simulink model "special_points"  (R2022b)
settings: Solver=VariableStepAuto  StartTime=0.0  StopTime=10  RelTol=1e-3
settings Model: Creator=Ivan  LastModifiedBy=anver
settings OptimizationCC: ReuseModelBlockBuffer=on

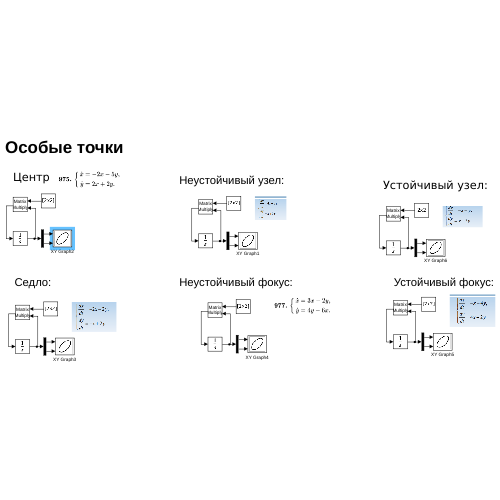
[thumbnail: Simulink's stored preview of the top-level diagram]
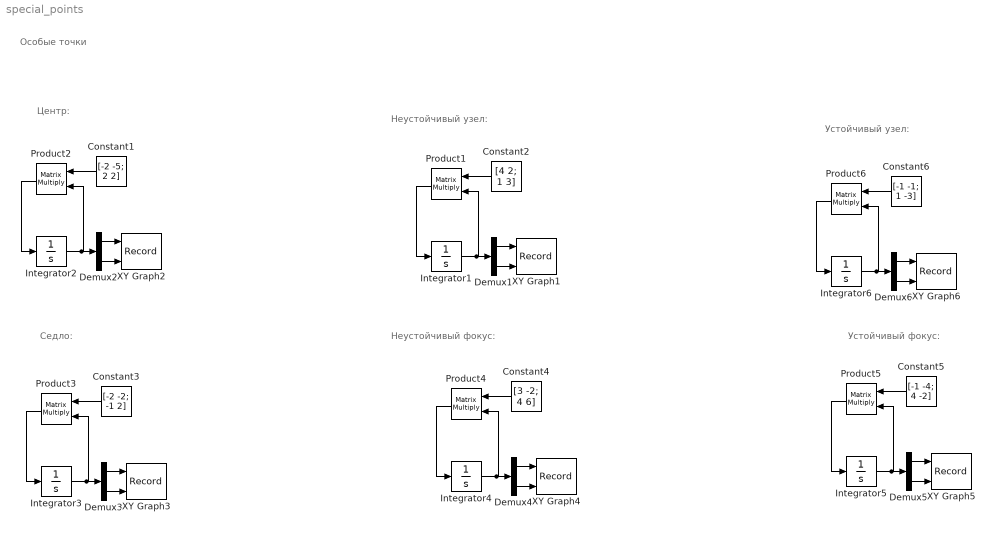
== system special_points ==
  note: Устойчивый узел:
  note: Седло:
  note: Центр:
  note: Особые точки
  note: Неустойчивый фокус:
  note: Неустойчивый узел:
  note: Устойчивый фокус:
  Constant1 : Constant  Value=[-2 -5; 2 2]
  Constant2 : Constant  Value=[4 2; 1 3]
  Constant3 : Constant  Value=[-2 -2; -1 2]
  Constant4 : Constant  Value=[3 -2; 4 6]
  Constant5 : Constant  Value=[-1 -4; 4 -2]
  Constant6 : Constant  Value=[-1 -1; 1 -3]
  Demux{1..6} (6 alike) : Demux  Outputs=2
  Integrator{1..6} (6 alike) : Integrator  InitialCondition=[1; 1]
  Product{1..6} (6 alike) : Product  Multiplication=Matrix(*)
  XY Graph1 : Record  FileSettingsInternal="{\"entries\":[{\"content\":{\"excelSettings\":{\"content\":{},\"type\":\"Streamout.ExcelSettings\"}},\"type\":\"Streamout.FileSettingStorage\",\"uuid\":\"b29d8a9c-392a-4fb2-98d1-ab0fd2f5d560\"}],\"packageUris\":[\"http://schema.mathworks.com/mf0/streamout_blocks/R2020a\"],\"version\":\"1.0\"}"  Layout=[1 1]  SignalsInternal="{\"entries\":[{\"content\":{\"signals\":[{\"content\":{\"blockPath\":[\"specialpoints/XY Graph1\"],\"channel\":[],\"dimensions\":[1],\"domain\":\"specialpoints/XY Graph1\",\"lineColor\":\"#a2142f\",\"plots\":[1],\"port\":1,\"sid\":[\"\"],\"signalID\":67,\"signalName\":\"Demux1:1\"},\"type\":\"RecordBlkView.Signal\",\"uuid\":\"e284521d-6ec3-49b5-a947-304f1478cd59\"},{\"content\":{\"blockPath\":[\"specialpoints/XY Graph1\"],\"channel\":[],\"dimensions\":[1],\"domain\":\"specialpoints/XY Graph1\",\"lineColor\":\"#139fff\",\"plots\":[1],\"port\":2,\"sid\":[\"\"],\"signalID\":71,\"signalName\":\"Demux1:2\"},\"type\":\"RecordBlkView.Signal\",\"uuid\":\"8df6b733-6354-4f83-b4f7-c70068da76a6\"}]},\"type\":\"RecordBlkView.InputSignals\",\"uuid\":\"bb9e6b20-75a7-4c07-86ad-f0d557820732\"}],\"packageUris\":[\"http://schema.mathworks.com/mf0/streamout_blocks/R2020a\"],\"version\":\"1.0\"}"  VisualizationBindings="{\"xyplotplugin\":{\"info\":[{\"series\":[{\"bindingParametersList\":[{\"parameter\":\"X-Axis\",\"signalID\":67,\"signalName\":\"Demux1:1\"},{\"parameter\":\"Y-Axis\",\"signalID\":71,\"signalName\":\"Demux1:2\"}],\"seriesID\":26685}],\"subplotID\":1}]}}"  CompatibilityTag=XY
  XY Graph2 : Record  FileSettingsInternal="{\"entries\":[{\"content\":{\"excelSettings\":{\"content\":{},\"type\":\"Streamout.ExcelSettings\"}},\"type\":\"Streamout.FileSettingStorage\",\"uuid\":\"a0532e12-d950-4453-bbc3-ca59d96ccae8\"}],\"packageUris\":[\"http://schema.mathworks.com/mf0/streamout_blocks/R2020a\"],\"version\":\"1.0\"}"  Layout=[1 1]  SignalsInternal="{\"entries\":[{\"content\":{\"signals\":[{\"content\":{\"blockPath\":[\"specialpoints/XY Graph2\"],\"channel\":[],\"dimensions\":[1],\"domain\":\"specialpoints/XY Graph2\",\"lineColor\":\"#a2142f\",\"plots\":[1],\"port\":1,\"sid\":[\"\"],\"signalID\":59,\"signalName\":\"Demux2:1\"},\"type\":\"RecordBlkView.Signal\",\"uuid\":\"02553b2b-631b-43a1-b492-2037fb39ac76\"},{\"content\":{\"blockPath\":[\"specialpoints/XY Graph2\"],\"channel\":[],\"dimensions\":[1],\"domain\":\"specialpoints/XY Graph2\",\"lineColor\":\"#139fff\",\"plots\":[1],\"port\":2,\"sid\":[\"\"],\"signalID\":63,\"signalName\":\"Demux2:2\"},\"type\":\"RecordBlkView.Signal\",\"uuid\":\"8bd99721-c510-42f4-8a47-9157c50785ae\"}]},\"type\":\"RecordBlkView.InputSignals\",\"uuid\":\"8468d6b2-b3e3-4423-a976-07fda8fce5e6\"}],\"packageUris\":[\"http://schema.mathworks.com/mf0/streamout_blocks/R2020a\"],\"version\":\"1.0\"}"  VisualizationBindings="{\"xyplotplugin\":{\"info\":[{\"series\":[{\"bindingParametersList\":[{\"parameter\":\"X-Axis\",\"signalID\":59,\"signalName\":\"Demux2:1\"},{\"parameter\":\"Y-Axis\",\"signalID\":63,\"signalName\":\"Demux2:2\"}],\"seriesID\":13331}],\"subplotID\":1}]}}"  CompatibilityTag=XY
  XY Graph3 : Record  FileSettingsInternal="{\"entries\":[{\"content\":{\"excelSettings\":{\"content\":{},\"type\":\"Streamout.ExcelSettings\"}},\"type\":\"Streamout.FileSettingStorage\",\"uuid\":\"69cbb6f6-f3a5-44cd-92ef-4036cbebcdd5\"}],\"packageUris\":[\"http://schema.mathworks.com/mf0/streamout_blocks/R2020a\"],\"version\":\"1.0\"}"  Layout=[1 1]  SignalsInternal="{\"entries\":[{\"content\":{\"signals\":[{\"content\":{\"blockPath\":[\"specialpoints/XY Graph3\"],\"channel\":[],\"dimensions\":[1],\"domain\":\"specialpoints/XY Graph3\",\"lineColor\":\"#a2142f\",\"plots\":[1],\"port\":1,\"sid\":[\"\"],\"signalID\":75,\"signalName\":\"Demux3:1\"},\"type\":\"RecordBlkView.Signal\",\"uuid\":\"47cecb95-6076-4ee7-86e1-f1b5dc16acf8\"},{\"content\":{\"blockPath\":[\"specialpoints/XY Graph3\"],\"channel\":[],\"dimensions\":[1],\"domain\":\"specialpoints/XY Graph3\",\"lineColor\":\"#139fff\",\"plots\":[1],\"port\":2,\"sid\":[\"\"],\"signalID\":79,\"signalName\":\"Demux3:2\"},\"type\":\"RecordBlkView.Signal\",\"uuid\":\"91964f3b-7724-463e-8b5d-57be4e640c57\"}]},\"type\":\"RecordBlkView.InputSignals\",\"uuid\":\"1ea9a202-36d1-423e-b5ef-d386424ed832\"}],\"packageUris\":[\"http://schema.mathworks.com/mf0/streamout_blocks/R2020a\"],\"version\":\"1.0\"}"  VisualizationBindings="{\"xyplotplugin\":{\"info\":[{\"series\":[{\"bindingParametersList\":[{\"parameter\":\"X-Axis\",\"signalID\":75,\"signalName\":\"Demux3:1\"},{\"parameter\":\"Y-Axis\",\"signalID\":79,\"signalName\":\"Demux3:2\"}],\"seriesID\":54321}],\"subplotID\":1}]}}"  CompatibilityTag=XY
  XY Graph4 : Record  FileSettingsInternal="{\"entries\":[{\"content\":{\"excelSettings\":{\"content\":{},\"type\":\"Streamout.ExcelSettings\"}},\"type\":\"Streamout.FileSettingStorage\",\"uuid\":\"88a36fd6-7621-4d16-9cb3-468432706825\"}],\"packageUris\":[\"http://schema.mathworks.com/mf0/streamout_blocks/R2020a\"],\"version\":\"1.0\"}"  Layout=[1 1]  SignalsInternal="{\"entries\":[{\"content\":{\"signals\":[{\"content\":{\"blockPath\":[\"specialpoints/XY Graph4\"],\"channel\":[],\"dimensions\":[1],\"domain\":\"specialpoints/XY Graph4\",\"lineColor\":\"#a2142f\",\"plots\":[1],\"port\":1,\"sid\":[\"\"],\"signalID\":83,\"signalName\":\"Demux4:1\"},\"type\":\"RecordBlkView.Signal\",\"uuid\":\"77b31cb0-8e9b-42f2-81eb-f84cb2f67803\"},{\"content\":{\"blockPath\":[\"specialpoints/XY Graph4\"],\"channel\":[],\"dimensions\":[1],\"domain\":\"specialpoints/XY Graph4\",\"lineColor\":\"#139fff\",\"plots\":[1],\"port\":2,\"sid\":[\"\"],\"signalID\":87,\"signalName\":\"Demux4:2\"},\"type\":\"RecordBlkView.Signal\",\"uuid\":\"21fa5dc8-c382-464e-aa4c-53efbbb9609e\"}]},\"type\":\"RecordBlkView.InputSignals\",\"uuid\":\"7114cbdf-c82f-41cb-8a52-ea1fd9a40c1c\"}],\"packageUris\":[\"http://schema.mathworks.com/mf0/streamout_blocks/R2020a\"],\"version\":\"1.0\"}"  VisualizationBindings="{\"xyplotplugin\":{\"info\":[{\"series\":[{\"bindingParametersList\":[{\"parameter\":\"X-Axis\",\"signalID\":83,\"signalName\":\"Demux4:1\"},{\"parameter\":\"Y-Axis\",\"signalID\":87,\"signalName\":\"Demux4:2\"}],\"seriesID\":54038}],\"subplotID\":1}]}}"  CompatibilityTag=XY
  XY Graph5 : Record  FileSettingsInternal="{\"entries\":[{\"content\":{\"excelSettings\":{\"content\":{},\"type\":\"Streamout.ExcelSettings\"}},\"type\":\"Streamout.FileSettingStorage\",\"uuid\":\"fc638fc8-ea17-4822-ae91-b9c87cfefd68\"}],\"packageUris\":[\"http://schema.mathworks.com/mf0/streamout_blocks/R2020a\"],\"version\":\"1.0\"}"  Layout=[1 1]  SignalsInternal="{\"entries\":[{\"content\":{\"signals\":[{\"content\":{\"blockPath\":[\"specialpoints/XY Graph5\"],\"channel\":[],\"dimensions\":[1],\"domain\":\"specialpoints/XY Graph5\",\"lineColor\":\"#a2142f\",\"plots\":[1],\"port\":1,\"sid\":[\"\"],\"signalID\":91,\"signalName\":\"Demux5:1\"},\"type\":\"RecordBlkView.Signal\",\"uuid\":\"b6c07a15-30d8-4ff6-8fc7-c4368179db7e\"},{\"content\":{\"blockPath\":[\"specialpoints/XY Graph5\"],\"channel\":[],\"dimensions\":[1],\"domain\":\"specialpoints/XY Graph5\",\"lineColor\":\"#139fff\",\"plots\":[1],\"port\":2,\"sid\":[\"\"],\"signalID\":95,\"signalName\":\"Demux5:2\"},\"type\":\"RecordBlkView.Signal\",\"uuid\":\"5dd7e6f7-038d-4159-a400-eb5585818727\"}]},\"type\":\"RecordBlkView.InputSignals\",\"uuid\":\"a808722b-0bd2-4d93-a2af-6840994ce530\"}],\"packageUris\":[\"http://schema.mathworks.com/mf0/streamout_blocks/R2020a\"],\"version\":\"1.0\"}"  VisualizationBindings="{\"xyplotplugin\":{\"info\":[{\"series\":[{\"bindingParametersList\":[{\"parameter\":\"X-Axis\",\"signalID\":91,\"signalName\":\"Demux5:1\"},{\"parameter\":\"Y-Axis\",\"signalID\":95,\"signalName\":\"Demux5:2\"}],\"seriesID\":12152}],\"subplotID\":1}]}}"  CompatibilityTag=XY
  XY Graph6 : Record  FileSettingsInternal="{\"entries\":[{\"content\":{\"excelSettings\":{\"content\":{},\"type\":\"Streamout.ExcelSettings\"}},\"type\":\"Streamout.FileSettingStorage\",\"uuid\":\"a1b310a2-b47b-471c-a264-dc29df9eae67\"}],\"packageUris\":[\"http://schema.mathworks.com/mf0/streamout_blocks/R2020a\"],\"version\":\"1.0\"}"  Layout=[1 1]  SignalsInternal="{\"entries\":[{\"content\":{\"signals\":[{\"content\":{\"blockPath\":[\"specialpoints/XY Graph6\"],\"channel\":[],\"dimensions\":[1],\"domain\":\"specialpoints/XY Graph6\",\"lineColor\":\"#a2142f\",\"plots\":[1],\"port\":1,\"sid\":[\"\"],\"signalID\":99,\"signalName\":\"Demux6:1\"},\"type\":\"RecordBlkView.Signal\",\"uuid\":\"7df400d1-39c8-4384-8a19-3b675b49f642\"},{\"content\":{\"blockPath\":[\"specialpoints/XY Graph6\"],\"channel\":[],\"dimensions\":[1],\"domain\":\"specialpoints/XY Graph6\",\"lineColor\":\"#139fff\",\"plots\":[1],\"port\":2,\"sid\":[\"\"],\"signalID\":103,\"signalName\":\"Demux6:2\"},\"type\":\"RecordBlkView.Signal\",\"uuid\":\"7f1c3162-d0a3-4495-a5b7-2a04c341ce80\"}]},\"type\":\"RecordBlkView.InputSignals\",\"uuid\":\"bcf530f1-92e4-4985-8ee1-9a7db29024fd\"}],\"packageUris\":[\"http://schema.mathworks.com/mf0/streamout_blocks/R2020a\"],\"version\":\"1.0\"}"  VisualizationBindings="{\"xyplotplugin\":{\"info\":[{\"series\":[{\"bindingParametersList\":[{\"parameter\":\"X-Axis\",\"signalID\":99,\"signalName\":\"Demux6:1\"},{\"parameter\":\"Y-Axis\",\"signalID\":103,\"signalName\":\"Demux6:2\"}],\"seriesID\":55209}],\"subplotID\":1}]}}"  CompatibilityTag=XY
  wires:
  Product1/1 -> Integrator1/1
  Integrator1/1 -> Product1/2, Demux1/1
  Demux1/1 -> XY Graph1/1
  Demux1/2 -> XY Graph1/2
  Constant2/1 -> Product1/1
  Demux2/2 -> XY Graph2/2
  Demux2/1 -> XY Graph2/1
  Integrator2/1 -> Product2/2, Demux2/1
  Constant1/1 -> Product2/1
  Product2/1 -> Integrator2/1
  Constant3/1 -> Product3/1
  Integrator3/1 -> Product3/2, Demux3/1
  Demux3/2 -> XY Graph3/2
  Demux3/1 -> XY Graph3/1
  Product3/1 -> Integrator3/1
  Product4/1 -> Integrator4/1
  Demux4/1 -> XY Graph4/1
  Constant4/1 -> Product4/1
  Integrator4/1 -> Product4/2, Demux4/1
  Demux4/2 -> XY Graph4/2
  Constant5/1 -> Product5/1
  Product5/1 -> Integrator5/1
  Demux5/1 -> XY Graph5/1
  Integrator5/1 -> Product5/2, Demux5/1
  Demux5/2 -> XY Graph5/2
  Demux6/2 -> XY Graph6/2
  Demux6/1 -> XY Graph6/1
  Integrator6/1 -> Product6/2, Demux6/1
  Constant6/1 -> Product6/1
  Product6/1 -> Integrator6/1
